simulink model "Sampling_Device"  (R2022b)
settings: Solver=VariableStepAuto  StartTime=0.0  StopTime=10.0  RelTol=1e-3
values from neighbouring files (symbols this model uses):
  J = 30    [Sampling_Device_init.m]
  rule = 1    [Sampling_Device_init.m]
  T = 20    [Sampling_Device_init.m]
  Ts = 0.25    [Sampling_Device_init.m]
  x0 = [0;0]    [Sampling_Device_init.m]
libraries: simulink x3
settings Model: Creator=Akash  LastModifiedBy=Akash

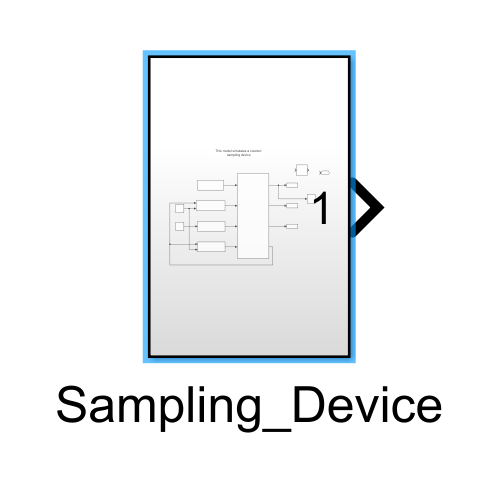
[thumbnail: Simulink's stored preview of the top-level diagram]
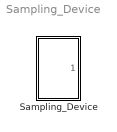
== system Sampling_Device ==
  Sampling_Device : Subsystem

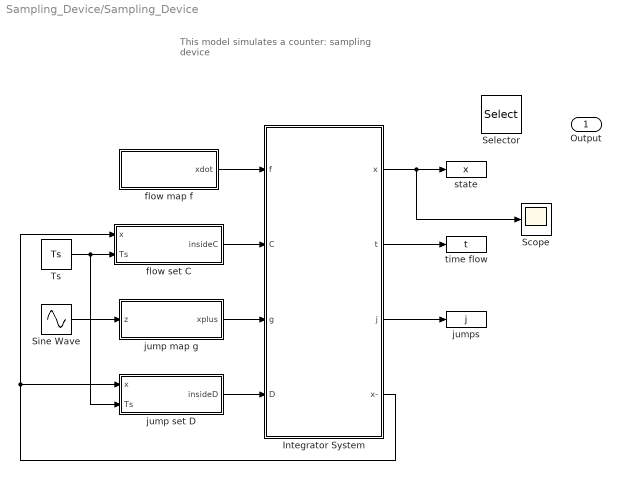
== system Sampling_Device/Sampling_Device ==
  note: This model simulates a counter: sampling device
  Integrator System : Subsystem  Priority=2  mask(Hybrid Integrator){T=T, J=J, x0=x0}
      mask prompts: T "Flow Horizon"; J "Jump Horizon"; x0 "Initial Condition"
      mask help:
      | This block integrates the state of the hybrid system defined by the flow map f (first input), the flow set C (second input), the jump map g (third input) and the jump set D (fourth input).
      | Starting from the initial condition x0 (last mask parameter), the system's state x evolves continuously within the set C, according to f(x,u), but is also subject to jumps within D, according to g(x,u).
      | The block also stops the simulation when the time t is greater than the flow horizon T (first mask parameter), or when the number of jumps j is greater than the jump horizon J (second mask parameter).
      | The outputs of the blocks are respectively x(t), t, j, x(t-).
      mask Help:
      | This block integrates the state of the hybrid system defined by the flow map f (first input), the flow set C (second input), the jump map g (third input) and the jump set D (fourth input).
      | <br>
      | Starting from the initial condition x0 (last mask parameter), the system's state x evolves continuously within the set C, according to f(x,u), but is also subject to jumps within D, according to g(x,u).
      | <br>
      | The block also stops the simulation when the time t is greater than the flow horizon T (first mask parameter), or when the number of jumps j is greater than the jump horizon J (second mask parameter).
      | <br>
      | The outputs of the blocks are respectively x(t), t, j, x(t-).
      | <br>
      | You can right click on the block and "Look under mask" to see what's inside the block.
      | Finally, refer to the manual (HybridSimulator_vXX.pdf) for more detailed information on how this hybrid simulator works.
  Scope : Scope
  Selector : Selector  NumberOfDimensions=2  InputPortWidth=3  IndexOptions=Index vector (dialog),Index vector (dialog)  Indices=1,1  OutputSizes=1,1
  Sine Wave : Sin  Amplitude=2  SampleTime=0
  Ts : Constant  Value=Ts
  flow map f : MATLAB Function  TreatAsAtomicUnit=on
  flow set C : MATLAB Function  TreatAsAtomicUnit=on
  jump map g : MATLAB Function  Priority=2  TreatAsAtomicUnit=on
  jump set D : MATLAB Function  TreatAsAtomicUnit=on
  jumps : ToWorkspace  VariableName=j  SampleTime=-1
  state : ToWorkspace  VariableName=x  SampleTime=-1
  "time flow " : ToWorkspace  VariableName=t  SampleTime=-1
  Output : Outport
  wires:
  Integrator System/4(x-) -> jump set D/1(x), flow set C/1(x)
  Ts/1 -> jump set D/2(Ts), flow set C/2(Ts)
  jump map g/1(xplus) -> Integrator System/3(g)
  Integrator System/1(x) -> Scope/1, state/1
  flow map f/1(xdot) -> Integrator System/1(f)
  Integrator System/3(j) -> jumps/1
  flow set C/1(insideC) -> Integrator System/2(C)
  Integrator System/2(t) -> "time flow "/1
  jump set D/1(insideD) -> Integrator System/4(D)
  Sine Wave/1 -> jump map g/1(z)

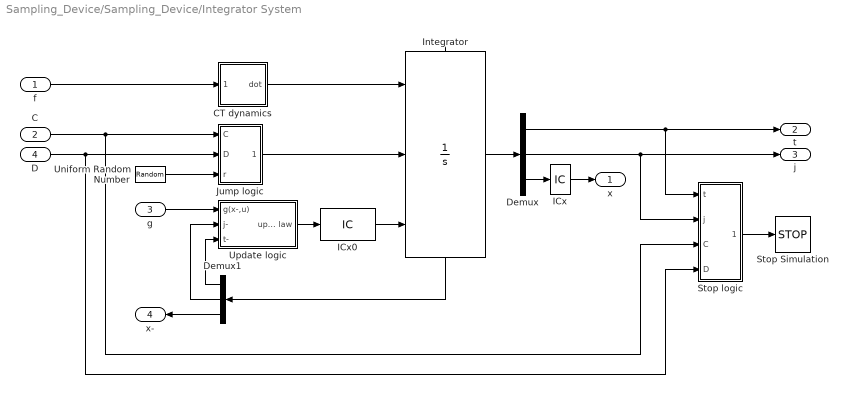
== system Sampling_Device/Sampling_Device/Integrator System ==
  f : Inport
  C : Inport  Port=2
  g : Inport  Port=3
  D : Inport  Port=4
  CT dynamics : Subsystem
  Demux : Demux  Outputs=[1 1 -1]
  Demux1 : Demux  Outputs=[1 1 -1]
  ICx : InitialCondition  Value=x0
  ICx0 : InitialCondition  Value=[0; 0; x0(:)]
  Integrator : Integrator  ExternalReset=level hold  InitialConditionSource=external  ShowStatePort=on  ZeroCross=off
  Jump logic : Subsystem
  Stop Simulation : Stop
  Stop logic : Subsystem
  Uniform Random Number : UniformRandomNumber  Minimum=0  Seed=abs(floor(100*rand))  SampleTime=0
  Update logic : Subsystem
  x : Outport  VectorParamsAs1DForOutWhenUnconnected=off
  t : Outport  Port=2  VectorParamsAs1DForOutWhenUnconnected=off
  j : Outport  Port=3  VectorParamsAs1DForOutWhenUnconnected=off
  x- : Outport  Port=4  VectorParamsAs1DForOutWhenUnconnected=off
  wires:
  Demux1/2 -> Update logic/2(j-)
  Demux1/1 -> Update logic/3(t-)
  g/1 -> Update logic/1(g(x-,u))
  Uniform Random Number/1 -> Jump logic/3(r)
  Jump logic/1(jump) -> Integrator/2
  Demux1/3 -> x-/1
  f/1 -> CT dynamics/1(f(x,u))
  D/1 -> Jump logic/2(D), Stop logic/4(D)
  C/1 -> Jump logic/1(C), Stop logic/3(C)
  Integrator/1 -> Demux/1
  CT dynamics/1(dot) -> Integrator/1
  Update logic/1(update law) -> ICx0/1
  Demux/1 -> Stop logic/1(t), t/1
  Demux/2 -> Stop logic/2(j), j/1
  Integrator/State -> Demux1/1
  Demux/3 -> ICx/1
  ICx/1 -> x/1
  ICx0/1 -> Integrator/3
  Stop logic/1(stop) -> Stop Simulation/1

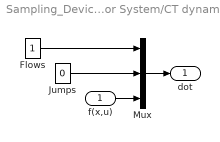
== system Sampling_Device/Sampling_Device/Integrator System/CT dynamics ==
  f(x,u) : Inport
  Flows : Constant
  Jumps : Constant  Value=0
  Mux : Mux  Inputs=[1 1 -1]
  dot : Outport  VectorParamsAs1DForOutWhenUnconnected=off
  wires:
  f(x,u)/1 -> Mux/3
  Mux/1 -> dot/1
  Flows/1 -> Mux/1
  Jumps/1 -> Mux/2

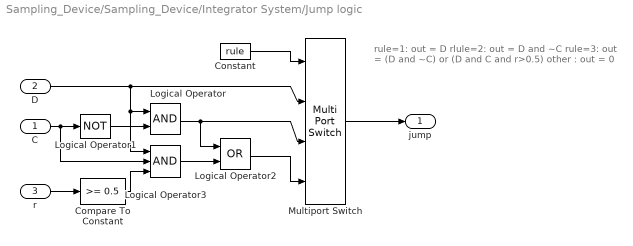
== system Sampling_Device/Sampling_Device/Integrator System/Jump logic ==
  note: rule=1:  out = D
      | rlule=2: out = D and ~C
      | rule=3:  out = (D and ~C)  or (D and C and r>0.5)
      | other :  out = 0
  C : Inport
  D : Inport  Port=2
  r : Inport  Port=3
  Compare To Constant : simulink/Logic and Bit Operations/Compare To Constant  relop=>=  const=0.5  OutDataTypeStr=uint8
  Constant : Constant  Value=rule
  Logical Operator : Logic  AllPortsSameDT=off  OutDataTypeStr=boolean
  Logical Operator1 : Logic  Operator=NOT  Inputs=1  AllPortsSameDT=off  OutDataTypeStr=boolean
  Logical Operator2 : Logic  Operator=OR  AllPortsSameDT=off  OutDataTypeStr=boolean
  Logical Operator3 : Logic  Inputs=3  AllPortsSameDT=off  OutDataTypeStr=boolean
  Multiport Switch : MultiPortSwitch  SaturateOnIntegerOverflow=off  InputSameDT=off
  jump : Outport  VectorParamsAs1DForOutWhenUnconnected=off
  wires:
  Logical Operator3/1 -> Logical Operator2/2
  Compare To Constant/1 -> Logical Operator3/3
  Multiport Switch/1 -> jump/1
  Logical Operator2/1 -> Multiport Switch/4
  Logical Operator/1 -> Logical Operator2/1, Multiport Switch/3
  Logical Operator1/1 -> Logical Operator/2
  C/1 -> Logical Operator1/1, Logical Operator3/2
  r/1 -> Compare To Constant/1
  D/1 -> Multiport Switch/2, Logical Operator/1, Logical Operator3/1
  Constant/1 -> Multiport Switch/1

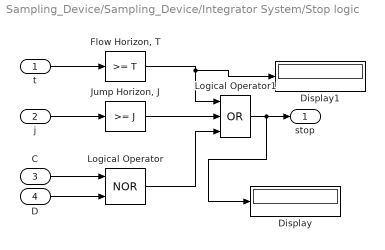
== system Sampling_Device/Sampling_Device/Integrator System/Stop logic ==
  t : Inport
  j : Inport  Port=2
  C : Inport  Port=3
  D : Inport  Port=4
  Display : Display
  Display1 : Display
  "Flow Horizon, T" : simulink/Logic and Bit Operations/Compare To Constant  relop=>=  const=T  OutDataTypeStr=uint8  ZeroCross=off
  "Jump Horizon, J" : simulink/Logic and Bit Operations/Compare To Constant  relop=>=  const=J  OutDataTypeStr=uint8  ZeroCross=off
  Logical Operator : Logic  Operator=NOR  AllPortsSameDT=off  OutDataTypeStr=boolean
  Logical Operator1 : Logic  Operator=OR  Inputs=3  AllPortsSameDT=off  OutDataTypeStr=boolean
  stop : Outport  VectorParamsAs1DForOutWhenUnconnected=off
  wires:
  Logical Operator1/1 -> Display/1, stop/1
  C/1 -> Logical Operator/1
  j/1 -> "Jump Horizon, J"/1
  t/1 -> "Flow Horizon, T"/1
  D/1 -> Logical Operator/2
  Logical Operator/1 -> Logical Operator1/3
  "Jump Horizon, J"/1 -> Logical Operator1/2
  "Flow Horizon, T"/1 -> Display1/1, Logical Operator1/1

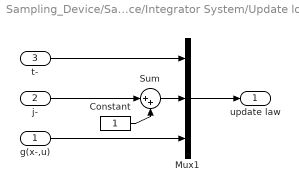
== system Sampling_Device/Sampling_Device/Integrator System/Update logic ==
  g(x-,u) : Inport
  j- : Inport  Port=2
  t- : Inport  Port=3
  Constant : Constant
  Mux1 : Mux  Inputs=[1 1 -1]
  Sum : Sum  Inputs=|++
  update law : Outport  VectorParamsAs1DForOutWhenUnconnected=off
  wires:
  Constant/1 -> Sum/2
  t-/1 -> Mux1/1
  g(x-,u)/1 -> Mux1/3
  j-/1 -> Sum/1
  Mux1/1 -> update law/1
  Sum/1 -> Mux1/2

== matlab function Sampling_Device/jump set D ==
  data: x input; insideD output; Ts input
function insideD = D_counter(x, Ts) 

%%%%%%%%%%%%%%%%%%%%%%%%%%%%%%%%%%%%%%%%%%%%%%%%%%%%%%%%%%%%%%%%%%%%%%%%%%%
% Matlab M-file             
% Project: Simulation of a counter
%
% Name: D_counter.m
%
% Description: Jump set
% Return 0 if outside of D, and 1 inside of D
%%%%%%%%%%%%%%%%%%%%%%%%%%%%%%%%%%%%%%%%%%%%%%%%%%%%%%%%%%%%%%%%%%%%%%%%%%%

%x = zeros(2,1)
%y = x

if (x(2) >= Ts || x(2) < 0)
    insideD = 1;
else 
    insideD = 0;
end

end

== matlab function Sampling_Device/flow map f ==
  data: xdot output
function xdot = f_counter

%%%%%%%%%%%%%%%%%%%%%%%%%%%%%%%%%%%%%%%%%%%%%%%%%%%%%%%%%%%%%%%%%%%%%%%%%%%
% Matlab Function 
% Project: Simulation of a counter
%
% Name: f_counter.m
%
% Description: Flow map
%
%%%%%%%%%%%%%%%%%%%%%%%%%%%%%%%%%%%%%%%%%%%%%%%%%%%%%%%%%%%%%%%%%%%%%%%%%%%

xdot = [0;1];
end

== matlab function Sampling_Device/flow set C ==
  data: x input; insideC output; Ts input
function insideC  = C_counter(x, Ts) 

%%%%%%%%%%%%%%%%%%%%%%%%%%%%%%%%%%%%%%%%%%%%%%%%%%%%%%%%%%%%%%%%%%%%%%%%%%%
% Matlab M-file             
% Project: Simulation of a counter
%
% Name: C_counter.m
%
% Description: Flow set
% Return 0 if outside of C, and 1 inside of C
%%%%%%%%%%%%%%%%%%%%%%%%%%%%%%%%%%%%%%%%%%%%%%%%%%%%%%%%%%%%%%%%%%%%%%%%%%%

x = zeros(2,1);
y = x;

if (y(2) >= 0) && (y(2) < Ts)  % flow condition
    insideC = 1;  % report flow
else
    insideC = 0;   % do not report flow
end
end

== matlab function Sampling_Device/jump map g ==
  data: xplus output; z input
function xplus = g_counter(z)

%%%%%%%%%%%%%%%%%%%%%%%%%%%%%%%%%%%%%%%%%%%%%%%%%%%%%%%%%%%%%%%%%%%%%%%%%%%
% Matlab Function
% Project: Simulation of a counter
%
% Name: g_coutner.m
%
% Description: Jump map
%
%%%%%%%%%%%%%%%%%%%%%%%%%%%%%%%%%%%%%%%%%%%%%%%%%%%%%%%%%%%%%%%%%%%%%%%%%%%

xplus = [z;0];
end
